simulink model "modelo_planta"  (R2023b)
settings: Solver=VariableStepAuto  StartTime=0.0  StopTime=inf  MaxStep=1e-3  RelTol=1e-3
undefined symbols (not defined in the file): ah_max, at_max, bcx, bcy, bhb, bhd, bhEb, bhm, bhwu, bt, btb, btd, btm, btw, DiscIntNeverNeededParam, g, h_vec_inicial, Hc, ih, it, J_hd_hEb, J_hm_hb, Jtd, Jtm_tb, Kcy, khwu, Ki_h, Ki_t, Kp_h, Kp_t, Kpos_h, Kpos_t, Ktw, lambda, Lh0, lh_0, magnitude, Mc_max, Mc_min, Ms, Mt, P_nom, rhd, rtd, tau_hm, tau_tm, Thb_Max, ThEb_Max, Thm_0, Thm_Max, titahm_0, titatm_0, Ts0, Ts1, Ts2, Ttb_Max, Ttm_0, Ttm_Max, vh_max_unloaded, vh_nom ... (+20)
libraries: simulink x14, vrlib x1, simulink_extras x1, dspnetwork x1
(part 2 of 2)

== stateflow chart modelo_planta/Control Nivel 1 ==
  settings: updateMethod=DISCRETE  sampleTime=Ts1
  state MAQUINA_ESTADOS [parallel]
    settings: executionOrder=1
    state AUTO
      state CICLO_SIMPLE
        entry:
        ciclo_doble = 0;
      state SELECCION_INDICE_INI_1
        entry:
        seleccionando_i(1) = 1;
        seleccionando = 1;
        is_cont = 0;
        during:
        i_ini1 = i_x_cruz;
        is_cont = check_container(i_ini1, yc0_vec);
        exit:
        i_obj_vec(1) = i_ini1;
        seleccionando_i(1) = 0;
      state SELECCION_INDICE_FIN_1
        entry:
        seleccionando_i(2) = 1;
        during:
        i_fin1 = i_x_cruz;
        exit:
        i_obj_vec(2) = i_fin1;
        seleccionando_i(2) = 0;
      state SELECCION_INDICE_INI_2
        entry:
        seleccionando_i(3) = 1;
        is_cont = 0;
        during:
        i_ini2 = i_x_cruz;
        is_cont = check_container(i_ini2, yc0_vec);
        exit:
        i_obj_vec(3) = i_ini2;
        seleccionando_i(3) = 0;
      state AUTO_INIT
        entry:
        modo_auto = 1; modo_manual = 0;
        BRK_t_N1 = 1; BRK_h_N1 = 1;
        x_cmd = 0; y_cmd = 0;
        estado = 1; % Bandera de etapa de movimiento
        i_obj_vec = [0,0,0,0];
        seleccionando_i = [0,0,0,0];
        modo_manual_auto = 0; flag = 0;
      state CICLO_DOBLE
        entry:
        ciclo_doble = 1;
      state SELECCION_INDICE_FIN_2
        entry:
        seleccionando_i(4) = 1;
        during:
        i_fin2 = i_x_cruz;
        exit:
        i_obj_vec(4) = i_fin1;
        seleccionando_i(4) = 0;
      state MANUAL_SIMPLE
        entry:
        modo_manual = 1; modo_auto = 0;
        modo_manual_auto = 1; flag = 0;
        y_handover = y_ref;
        y_cruz = y_ref;
        x_cruz = x_ref;
        during:
        x_cruz = xt_enc;
        y_ref = y_cruz;
        if (TLK == 0)
        y_cruz = max([yc0-offset, min(y_handover, y_cruz)]);
        elseif (TLK == 1)
        y_cruz = max([(yc0+Hc)-offset, min(y_handover, y_cruz)]);
        end
        exit:
        estado = estado + 1;
      state MOVIMIENTO_CURVO
        entry:
        modo_auto = 1;
        modo_manual_auto = 0; flag = 1;
        manual_ok = 0;
        i_usado = 0;
        seleccionando = 0;
        during:
        if (estado == 1) i_usado = i_ini1;
        elseif (estado == 2) i_usado = i_fin1;
        elseif (estado == 3) i_usado = i_ini2;
        elseif (estado == 4) i_usado = i_fin2;
        end
        [x_cmd, y_cmd, manual_ok] = Planificador_Trayectoria...
        (xt_enc, yh_enc, i_usado, yc0_vec, TLK, theta_l);
        x_ref = x_cmd;
        y_ref = y_cmd;
        % Actualizar cruz con referencias
        x_cruz = x_ref;
        y_cruz = y_ref;
      (default) -> MAQUINA_ESTADOS.AUTO.AUTO_INIT
      CICLO_SIMPLE -> MAQUINA_ESTADOS.AUTO.SELECCION_INDICE_INI_1 [order 1] : [rising(BTN_TLK)]
      MAQUINA_ESTADOS.AUTO.AUTO_INIT -> CICLO_SIMPLE
      CICLO_SIMPLE -> CICLO_DOBLE [order 2] : [rising(BTN_Auto)]
      CICLO_DOBLE -> CICLO_SIMPLE [order 2] : [rising(BTN_Auto)]
      MAQUINA_ESTADOS.AUTO.SELECCION_INDICE_INI_1 -> MAQUINA_ESTADOS.AUTO.SELECCION_INDICE_FIN_1 : [rising(BTN_TLK)&& is_cont == 1]
      MAQUINA_ESTADOS.AUTO.SELECCION_INDICE_FIN_1 -> SELECCION_INDICE_INI_2 [order 2] : [rising(BTN_TLK) && ciclo_doble == 1]
      CICLO_DOBLE -> MAQUINA_ESTADOS.AUTO.SELECCION_INDICE_INI_1 [order 1] : [rising(BTN_TLK)]
      MAQUINA_ESTADOS.AUTO.SELECCION_INDICE_FIN_1 -> MOVIMIENTO_CURVO [order 1] : [rising(BTN_TLK) && ciclo_doble == 0]
      MANUAL_SIMPLE -> MAQUINA_ESTADOS.AUTO.AUTO_INIT [order 1] : [TLK == 0 && yh_enc >= (y_handover - 0.1) && estado == 2 && ciclo_doble == 0]
      MANUAL_SIMPLE -> MAQUINA_ESTADOS.AUTO.AUTO_INIT [order 4] : [TLK == 0 && yh_enc >= (y_handover - 0.1) && estado == 4 && ciclo_doble == 1]
      SELECCION_INDICE_INI_2 -> SELECCION_INDICE_FIN_2 : [rising(BTN_TLK) && is_cont == 1 ]
      SELECCION_INDICE_FIN_2 -> MOVIMIENTO_CURVO : [rising(BTN_TLK)]
      MOVIMIENTO_CURVO -> MANUAL_SIMPLE [order 1] : [manual_ok == 1]
      MANUAL_SIMPLE -> MOVIMIENTO_CURVO [order 5] : [TLK == 1 && yh_enc >= (y_handover - 0.1) && estado == 3]
      MANUAL_SIMPLE -> MOVIMIENTO_CURVO [order 3] : [TLK == 0 && yh_enc >= (y_handover - 0.1) && estado == 2]
      MANUAL_SIMPLE -> MOVIMIENTO_CURVO [order 2] : [TLK == 1 && yh_enc >= (y_handover - 0.1) && estado == 1]
    state STOP
      entry:
      x_ref = xt_0; y_ref = yh_0;
      x_cruz = x_ref; y_cruz = y_ref;
      x_cruz_unity = x_ref; y_cruz_unity = y_ref;
      seleccionando = 0;
      vx_cmd = 0; vy_cmd = 0;
      BRK_t_N1 = 0; BRK_h_N1 = 0; % Frenos Cerrados
      modo_manual = 0; modo_auto = 0;
      dead_zone = 0.1; % Zona muerta joystick
      offset = 0.2; % Offset del apoyo
      modo_manual_auto = 0; flag = 0; % Bandera para bumpless transfer
      ciclo_doble = 0;
    state POSICION_SEGURA
      entry:
      x_ref = xt_0; y_ref = yh_0;
      BRK_t_N1 = 1; BRK_h_N1 = 1;
    state ERROR
      entry:
      BRK_t_N1 = 0; BRK_h_N1 = 0;
    state MANUAL
      state MANUAL_INIT [parallel]
        entry:
        % Si quiero mover, abro frenos
        BRK_t_N1 = 1;
        BRK_h_N1 = 1;
        modo_manual = 1;
        settings: executionOrder=1
      state INTEGRACION_JOYSTICK [parallel]
        during:
        % Copiar los movimientos de la cruceta
        x_ref = x_cruz
        y_ref = y_cruz
        % Cuando los índices son diferentes
        if(i_xt_ref ~= i_carro && y_ref<yc0_xtref+1)
        if (TLK == 1)
        y_ref = max([(yc0+Hc)-offset, (yc0_xtref+Hc)+1, min(yh_max, y_ref)]);
        else
        y_ref = max([yc0-offset, yc0_xtref+1, min(yh_max, y_ref)]);
        end
        % Aplico la limitación a la cruceta
        y_cruz = y_ref;
        % Cuando están en el mismo índice
        else
        if (TLK == 1)
        y_ref = max([(yc0+Hc)-offset, min(yh_max, y_ref)]);
        if (sobrecarga == 1)
        % No se puede mover en horizontal
        x_ref = xt_enc;
        % En vertical solo puede moverse hacia abajo
        y_ref = max([(yc0+Hc)-offset, min((yc0+Hc)+offset,y_ref)]);
        end
        else
        y_ref = max([yc0-offset, min(yh_max, y_ref)]);
        end
        end
        % Aplico las limitaciones del modo manual a la cruceta
        x_cruz = x_ref;
        y_cruz = y_ref;
        settings: executionOrder=2
    (default) -> STOP
    STOP -> AUTO [order 1] : [rising(BTN_Auto) && FALLA == 0]
    STOP -> ERROR [order 2] : [FALLA == 1]
    STOP -> MANUAL [order 3] : [rising(BTN_Manual) && FALLA == 0]
    POSICION_SEGURA -> STOP : [abs(xt_enc - x_ref) <= 0.1 && abs(yh_enc - y_ref) <= 0.1 && abs(vt_enc) <= 0.008]
    ERROR -> POSICION_SEGURA : [FALLA == 0 && rising(BTN_Reset)]
    AUTO -> ERROR [order 2] : [FALLA == 1]
    MANUAL -> ERROR [order 1] : [FALLA ==1 || FC_der == 1 || FC_izq == 1 || FC_sup == 1 || FC_inf == 1]
    AUTO -> MANUAL [order 1] : [rising(BTN_Manual) && modo_manual_auto == 0]
    MANUAL -> AUTO [order 3] : [rising(BTN_Auto) && flag == 0]
    MANUAL_SIMPLE -> MANUAL [order 6] : [rising(BTN_Manual) && modo_auto == 0]
    MANUAL -> MOVIMIENTO_CURVO [order 2] : [rising(BTN_Auto) && flag == 1]
    MOVIMIENTO_CURVO -> MANUAL [order 2] : [Joy_XY(1) > dead_zone || Joy_XY(2) > dead_zone || rising(BTN_Manual)]
  state MONITOREO_FISICO [parallel]
    settings: executionOrder=2
    state LIMITE_VEL_CARRO [parallel]
      during:
      factor_x = 1.0;
      dist_dinamica = 3.5 - (0.166 * yh_enc); % Definir zona de frenado (m antes del tope)
      dist_frenado_x = max(2.0, min(3.5, dist_dinamica)); % Saturación por seguridad (2m < x < 10m)
      % Acercándose al Muelle (xt_min)
      if (xt_enc < (xt_min + dist_frenado_x)) && (vx_cmd <= 0)
      factor_x = 0.1;  % 10% de la velocidad
      % Acercándose al Barco (xt_max)
      elseif (xt_enc > (xt_max - dist_frenado_x)) && (vx_cmd >= 0)
      factor_x = 0.1;
      end
      vt_lim = vt_max * factor_x;
      settings: executionOrder=1
    state TWISTLOCKS [parallel]
      settings: executionOrder=2
      state ABRIENDO_TLK
        entry:
        TLK = 0;
        y_start = yh_enc;
        trans_TLK = 1;
        during:
        vh_lim = 0.5;
        m_est = max(Ms, Fhw * 2 / g);
        y_ref = yh_enc + 0.5;
        x_ref = xt_enc;
        % Coordinar cruz con referencias
        y_cruz = y_ref;
        x_cruz = x_ref;
      state VACIO
        entry:
        TLK = 0;
        m_est = Ms;
        vh_lim = vh_max_unloaded;
        sobrecarga = 0;
        trans_TLK = 0;
      state CERRANDO_TLK
        entry:
        TLK = 1;
        y_start = yh_enc;
        trans_TLK = 1;
        during:
        vh_lim = 0.5;
        m_est = max(Ms, (Fhw * 2 / g));
        y_ref = yh_enc + 0.1;
        x_ref = xt_enc;
        % Coordinar cruz con referencias
        y_cruz = y_ref;
        x_cruz = x_ref;
      state CARGADO
        entry:
        trans_TLK = 0;
        v_potencia = P_nom / (m_est * g);
        vh_lim = min(vh_max_unloaded, max(vh_nom, v_potencia));
        % Sobrecarga (margen 100kg)
        if (m_est > (Ms + Mc_max + 100))
        sobrecarga = 1;
        vh_lim = 0.1;
        vt_lim = 0;
        end
        during:
        m_est = max(Ms, (Fhw * 2 / g));
      (default) -> VACIO
      ABRIENDO_TLK -> VACIO : [Fhw >= (Ms*g/2*0.8) && (yh_enc - y_start) > 0.3 &&  xt_enc <= x_ref + 0.1]
      VACIO -> CERRANDO_TLK : [rising(BTN_TLK) == 1 && Fhw < (Ms*g/2*0.8) && ((i_carro<13 && yc0>0 ) || (i_carro>13 && i_carro<33 && yc0>-18))]
      CARGADO -> ABRIENDO_TLK : [falling(BTN_TLK) == 1 && Fhw < (m_est*g/2*0.8)]
      CERRANDO_TLK -> CARGADO : [Fhw > (Ms*g/2 * 1.2) && (yh_enc - y_start) > 0.3 && xt_enc <= x_ref +0.1]
  state MODO_AUTO_CUADRADO [parallel] [commented out]
    state AUTO_INIT [commented out]
      entry:
      modo_auto = 1; modo_manual = 0;
      BRK_t_N1 = 1; BRK_h_N1 = 1;
      x_cmd = 0; y_cmd = 0;
      flag = 0;
    state SELECCION_INDICE_FIN_1 [commented out]
      entry:
      i_fin1 = 20;
      exit:
      flag = 1;
    state SELECCION_INDICE_INI_1 [commented out]
      entry:
      i_ini1 = 5;
      ini = check_container(i_ini1, yc0_vec);
    state MODO_MANUAL [commented out]
      entry:
      modo_manual = 1;
      v_max_ref = 3;     % Vel. de la referencia
      y_handover = y_ref;
      during:
      Joy_CMD_Y = Joy_XY(2);
      if abs(Joy_CMD_Y) < dead_zone
      vy_cmd = 0;
      else
      vy_cmd = Joy_CMD_Y * v_max_ref;
      end
      y_ref = y_ref + vy_cmd * Ts1;
      if (TLK == 0)
      y_ref = max([yc0-offset, min(y_handover, y_ref)]);
      elseif (TLK == 1)
      y_ref = max([(yc0+Hc)-offset, min(y_handover, y_ref)]);
      end
      exit:
      modo_auto = modo_auto + 1;
    state BUSCAR_Y_MOVER_Y1 [commented out]
      entry:
      BRK_t_N1 = 1; BRK_h_N1 = 1;
      if modo_auto == 0
      if i_carro < i_ini1
      max_h = max(yc0_vec(i_carro : i_ini1));
      else
      max_h = max(yc0_vec(i_ini1 : i_carro));
      end
      y_ref = max_h + 2; % 2m de h_max
      elseif modo_auto == 1
      if i_carro < i_fin1
      max_h = max(yc0_vec(i_carro : i_fin1));
      else
      max_h = max(yc0_vec(i_fin1 : i_carro));
      end
      y_ref = max_h + 2 + Hc; % 2m de h_max
      end
    state MOVER_X1 [commented out]
      entry:
      if modo_auto == 0
      if i_carro < i_ini1
      x_ref = xt_min + (i_ini1-1) * Wc - Wc/2;
      elseif i_carro > i_ini1
      x_ref = xt_min + (i_ini1+1) * Wc - Wc/2;
      end
      elseif modo_auto == 1
      if i_carro < i_fin1
      x_ref = xt_min + (i_fin1-2) * Wc - Wc/2;
      elseif i_carro > i_fin1
      x_ref = xt_min + (i_fin1+2) * Wc - Wc/2;
      end
      end
    state BAJAR_SPREADER1 [commented out]
      entry:
      if modo_auto == 0
      y_ref = yc0_vec(i_ini1) + 2;
      elseif modo_auto == 1
      y_ref = (yc0_vec(i_fin1) + Hc) +2
      end
      y_handover = y_ref;
    state MOVER_X2 [commented out]
      entry:
      if modo_auto == 0
      x_ref = xt_min + i_ini1 * Wc - Wc/2;
      elseif modo_auto == 1
      x_ref = xt_min + i_fin1 * Wc - Wc/2;
      end
    (default) -> MODO_AUTO_CUADRADO.AUTO_INIT [commented out]
    MODO_AUTO_CUADRADO.SELECCION_INDICE_INI_1 -> MODO_AUTO_CUADRADO.SELECCION_INDICE_FIN_1 [commented out] : [rising(BTN_Auto) && ini == 1]
    MODO_AUTO_CUADRADO.AUTO_INIT -> MODO_AUTO_CUADRADO.SELECCION_INDICE_INI_1 [commented out] : [rising(BTN_Auto)]
    MODO_AUTO_CUADRADO.SELECCION_INDICE_FIN_1 -> BUSCAR_Y_MOVER_Y1 [commented out] : [rising(BTN_Auto)]
    MODO_MANUAL -> MODO_AUTO_CUADRADO.AUTO_INIT [commented out] : [TLK == 0 && yh_enc >= (y_handover - 0.1) && modo_auto == 2]
    MODO_MANUAL -> BUSCAR_Y_MOVER_Y1 [commented out] : [TLK == 1 && yh_enc >= (y_handover - 0.1) && modo_auto == 0]
    BUSCAR_Y_MOVER_Y1 -> MOVER_X1 [commented out] : [yh_enc > y_ref || abs(yh_enc - y_ref) <= 3]
    BAJAR_SPREADER1 -> MODO_MANUAL [commented out] : [abs(yh_enc - y_ref) <= 0.1]
    MOVER_X2 -> BAJAR_SPREADER1 [commented out] : [abs(xt_enc - x_ref) <= 0.1]
    MOVER_X1 -> MOVER_X2 [commented out] : [abs(xt_enc - x_ref) <= 2]
  state INIDICES_Y_PERFIL [parallel]
    settings: executionOrder=3
    state ACTUALIZAR_PERFIL_ALTURAS [parallel]
      entry:
      yc0_xtref = 0;
      yc0 = 0;
      yc0_vec_output = yc0_vec;
      h_vec_output = h_vec;
      TLK_anterior = 0;
      during:
      yc0_xtref = yc0_vec(i_xt_ref); % Obtengo altura donde esta la referencia
      yc0_vec_output(i_lidar) = h_vec(i_lidar); % Actualizo perfil con la medición real
      %Detecto si se ha abierto o cerrado TLK
      TLK_rise  = (TLK_anterior == 0) && (TLK == 1);
      TLK_fall  = (TLK_anterior == 1) && (TLK == 0);
      % Si agarré un container, hay que bajar el perfil
      if(TLK_rise)
      h_vec_output(i_carro) = h_vec(i_carro)-Hc;
      yc0_vec_output(i_carro) = yc0_vec(i_carro)-Hc;
      %Si solté un container, hay que aumentar el perfil
      elseif(TLK_fall)
      h_vec_output(i_carro) = h_vec(i_carro)+Hc;
      yc0_vec_output(i_carro) = yc0_vec(i_carro)+Hc;
      end
      yc0 = yc0_vec_output(i_carro);
      TLK_anterior = TLK;
      settings: executionOrder=2
    state CALCULO_INDICES [parallel]
      entry:
      i_carro = 0;
      i_lidar = 0;
      i_xt_ref = 0;
      i_x_cruz = 0;
      during:
      i_carro = floor((xt_enc - xt_min)/Wc) + 1;
      i_carro = min(max(i_carro, 1), 33);
      i_lidar = floor((xt_enc+x_LIDAR-xt_min)/Wc)+1;
      i_lidar = min(max(i_lidar,1),33);
      i_xt_ref = floor((x_ref - xt_min)/Wc) + 1;
      i_xt_ref = min(max(i_xt_ref, 1), 33);
      i_x_cruz = floor((x_cruz - xt_min)/Wc) + 1;
      i_x_cruz = min(max(i_x_cruz, 1), 33);
      settings: executionOrder=1
  state HAY_CONTAINER_ABAJO [parallel] [commented out]
    entry:
    hay_container = 0;
    during:
    if(i_carro<13 && yc0>0)
    hay_container = 1;
    elseif(i_carro>13 && i_carro<33 &&yc0>-18)
    hay_container = 1;
    else
    hay_container=0;
    end
  note: El orden es importante! Si no van en orden los bloques no funcionan:
      | Maquina estados
      | Monitoreo fisico
      | Indices y perfil (¡siempre al último!)
  state MANEJO_CRUCETA [parallel]
    settings: executionOrder=4
    state INPUT_JOYSTICK [parallel]
      entry:
      v_max_ref = 8;     % Vel. de la referencia
      during:
      Joy_CMD_X = Joy_XY(1);
      Joy_CMD_Y = Joy_XY(2);
      if abs(Joy_CMD_X) < dead_zone
      vx_cmd = 0;
      else
      vx_cmd = Joy_CMD_X * v_max_ref;
      end
      if abs(Joy_CMD_Y) < dead_zone
      vy_cmd = 0;
      else
      vy_cmd = Joy_CMD_Y * v_max_ref;
      end
      if (trans_TLK == 1)
      vx_cmd = 0;
      vy_cmd = 0;
      end
      settings: executionOrder=1
    state ACTUALIZAR_CRUCETA [parallel]
      during:
      % Actualizar posición x de la cruceta
      x_cruz = x_cruz + vx_cmd * Ts1;
      % Actualizar posición y de la cruceta
      y_cruz = y_cruz + vy_cmd * Ts1;
      % Limitar en x
      x_cruz = max(xt_min, min(xt_max, x_cruz));
      % Limitar en y
      y_cruz = max(yh_min, min(yh_max, y_cruz));
      if seleccionando == 0
      x_cruz_unity = x_cruz;
      y_cruz_unity = y_cruz;
      else
      x_cruz_unity = xt_min + i_x_cruz * Wc - Wc/2;
      y_cruz_unity = yh_min;
      end
      settings: executionOrder=2
  data: i_pos function_input; y0_vec function_input; hay_container function_output; x_real function_input; y_real function_input; i_ref function_input; y0_vec function_input; twistlock function_input; tita_l function_input; x_ref_out function_output; y_ref_out function_output; listo_para_manual function_output; xt_enc function_input; yh_enc function_input; i_xt_ref function_input; h_vec function_input; TLK function_input; x_ref_out function_output; y_ref_out function_output; listo_para_manual function_output; vt_enc input; Fhw input size=1; BTN_TLK input size=1; m_est output size=1; vh_lim output size=1; vh_max_unloaded parameter size=1; P_nom parameter size=1; g parameter size=1; Ms parameter size=1; Joy_XY input; BTN_Manual input size=1; BTN_Auto input size=1; BTN_Reset input size=1; FC_der input size=1; FC_sup input size=1; FC_izq input size=1; FC_inf input size=1; xt_enc input size=1; yh_enc input size=1; FALLA input size=1; x_ref output size=1; y_ref output size=1; BRK_h_N1 output size=1; BRK_t_N1 output size=1; Ts1 parameter size=1; xt_0 parameter size=1; yh_0 parameter size=1; xt_max parameter size=1; xt_min parameter size=1; yh_max parameter size=1; vt_max parameter size=1; vt_lim output size=1; vh_nom parameter size=1; Mc_max parameter size=1; TLK output size=1; Wc parameter; x_LIDAR parameter; yc0 output; Hc parameter; yc0_vec input; yc0_vec_output output; h_vec input; h_vec_output output; i_fin1 local; i_xt_ref local; TLK_rise local; TLK_fall local; i_lidar local; y_start local; i_carro local; x_cmd local; y_cmd local; dist_dinamica local; dist_frenado_x local; trans_TLK local; sobrecarga local; yc0_xtref local; TLK_anterior local; v_potencia local; v_max_ref local; Joy_CMD_Y local; Joy_CMD_X local; dead_zone local; factor_x local; vx_cmd local; i_ini1 local; vy_cmd local; offset local; manual_ok local; y_handover local; flag local; i_fin2 local; i_ini2 local; i_usado local; modo_manual_auto local; modo_manual output; modo_auto output; theta_l input; estado local; ciclo_doble output; yh_min parameter; i_x_cruz local; is_cont local; seleccionando_i output; i_obj_vec output; seleccionando local; y_cruz local; x_cruz local; x_cruz_unity output; y_cruz_unity output
  function hay_container  = check_container(i_pos, y0_vec):
    | function hay_container  = check_container(i_pos, y0_vec)
    |    if(i_pos<13 && y0_vec(i_pos)>0)
    |        hay_container = 1;
    |    elseif(i_pos>13 && i_pos<33 && y0_vec(i_pos)>-18)
    |        hay_container = 1;
    |    else
    |        hay_container = 0;
    |    end
    | end
  function [x_ref_out, y_ref_out, listo_para_manual] = Planificador_Trayectoria...:
    | function [x_ref_out, y_ref_out, listo_para_manual] = Planificador_Trayectoria...
    |     (x_real, y_real, i_ref, y0_vec, twistlock, tita_l)
    |     
    |     % 1. SISTEMA DE MEMORIA (LATCH / HISTÉRESIS)
    |     % Estas variables recuerdan el estado entre ejecuciones para evitar
    |     % comportamientos erráticos ("twitching") cuando las señales oscilan en el umbral.
    |     persistent fase_final_latched; % Flag: true = yendo al objetivo real, false = esperando en objetivo falso
    |     persistent last_target_idx;    % Memoria del último destino solicitado por el usuario
    |     
    |     % Inicialización en el primer ciclo de reloj
    |     if isempty(fase_final_latched)
    |         fase_final_latched = false;
    |         last_target_idx = -1;
    |     end
    |     
    |     % RESETEO DE ESTADO:
    |     % Si el operador cambia el destino (ej. de índice 16 a 20),
    |     % forzamos el reinicio de la lógica de aproximación.
    |     if i_ref ~= last_target_idx
    |         fase_final_latched = false;
    |         last_target_idx = i_ref;
    |     end
    | 
    |     % 2. CONFIGURACIÓN Y PARÁMETROS DE SEGURIDAD
    |     % Márgenes geométricos para evitar colisiones físicas
    |     MARGEN_Y_SEG = 2.5;        % Altura extra sobre obstáculos durante el viaje
    |     MARGEN_HOVER = 2.5;        % Altura final sobre el objetivo (punto de entrega)
    |     GAP_X_SEGURIDAD = 1.5;     % Distancia de frenado antes de chocar lateralmente
    |     PENDIENTE_SUBIDA = 0.25;   % Relación de ascenso (1 m subida cada 4 m avance)
    |     
    |     % Definimos una ventana para la estabilidad del péndulo.
    |     % Para entrar a la zona de precisión, el ángulo debe ser muy bajo (< 1.0°)
    |     % Para salir (abortar), el ángulo debe ser muy alto (> 2.0°)
    |     % Esto evita que el sistema oscile entre modos si la variación del ángulo es pequeña.
    |     UMBRAL_ENTRADA = 0.0175; % ~1.0 grado
    |     UMBRAL_SALIDA  = 0.0349; % ~2.0 grados
    |     
    |     % COMPENSACIÓN DE ALTURA DE CARGA
    |     % Si llevamos contenedor (TLK=1), todo el sistema debe subir más
    |     % para compensar la altura física del objeto colgado (Hc).
    |     if twistlock == 1
    |         H_extra = Hc; 
    |     else
    |         H_extra = 0;  % Spreader vacío
    |     end
    |     
    |     % 3. MAPEO Y GESTIÓN DE OBJETIVOS
    |     N = length(y0_vec); 
    |     i_objetivo_final = i_ref;
    |     
    |     % Conversión: Posición actual (metros) -> Índice del mapa
    |     i_actual = floor((x_real - xt_min)/Wc) + 1;
    |     i_actual = min(max(i_actual, 1), N); % Saturación para no salir del vector
    |     
    |     % --- ESTRATEGIA DE OBJETIVO FALSO (ANTI-SWAY) ---
    |     % Definimos un "punto de espera" antes del destino real.
    |     % La grúa viajará rápido hasta aquí y esperará a que el balanceo se disipe.
    |     L_cable = 40.0 - y_real;
    |     
    |     % DIST_TRIGGER Dinámico 
    |     DIST_TRIGGER = 0.1 * L_cable; % Metros antes del objetivo falso para evaluar transición
    |     
    |     % Saturación para seguridad
    |     DIST_TRIGGER = max(0.1, min(5.0, DIST_TRIGGER));
    |     
    |     offset_idx = 1;   % Cantidad de celdas de anticipación
    |     
    |     % Determinar dirección de movimiento para saber de qué lado poner el falso
    |     dir_mov = sign(i_objetivo_final - i_actual);
    |     if dir_mov == 0, dir_mov = 1; end
    |     
    |     i_target_falso = i_objetivo_final - (dir_mov * offset_idx);
    |     
    |     % Cálculo del centro físico (en metros) del objetivo falso
    |     x_falso_m = xt_min + i_target_falso * Wc - Wc/2;
    |     
    |     % 4. LÓGICA DE TRANSICIÓN DE ESTADOS (MAQUINA DE ESTADOS)
    |     
    |     % A. Verificación de posición: ¿Ya llegamos al punto de trigger?
    |     distancia_ok = false;
    |     if dir_mov > 0 % Viajando a derecha
    |         if x_real >= (x_falso_m - DIST_TRIGGER)
    |             distancia_ok = true;
    |         end
    |     else % Viajando a izquierda
    |         if x_real <= (x_falso_m + DIST_TRIGGER)
    |             distancia_ok = true;
    |         end
    |     end
    |     
    |     % B. Lógica del Latch (Cerrojo)
    |     if fase_final_latched == false
    |         % ESTADO: APROXIMACIÓN (Viajando al objetivo falso)
    |         % Solo permitimos pasar a la fase final si estamos cerca Y el péndulo está quieto.
    |         if distancia_ok && (abs(tita_l) < UMBRAL_ENTRADA)
    |             fase_final_latched = true;
    |         end
    |     else
    |         % ESTADO: FASE FINAL (Posicionamiento fino en objetivo real)
    |         % Ya estamos comprometidos. Solo abortamos si la oscilación se vuelve peligrosa.
    |         if abs(tita_l) > UMBRAL_SALIDA
    |             fase_final_latched = false; % Abortar maniobra, volver a esperar
    |         end
    |     end
    | 
    |     % C. Selección de Referencia según el estado del Latch
    |     if fase_final_latched
    |         i_target_eff = i_objetivo_final; % Ir al hueco final
    |         fase_aproximacion = false; 
    |     else
    |         i_target_eff = i_target_falso;   % Quedarse esperando afuera
    |         fase_aproximacion = true;  
    |     end
    |     
    |     % Conversión final Índice -> Metros para el controlador de posición
    |     x_target_cmd = xt_min + i_target_eff * Wc - Wc/2;
    |     
    |     % 5. GENERACIÓN DE TRAYECTORIA SEGURA
    |     x_ref_out = x_target_cmd; 
    |     
    |     % PARTE A: ESCANEO DE PAREDES (BLOQUEO DE MOVIMIENTO X)
    |     % Proyectamos una diagonal desde la posición actual. Si algún obstáculo
    |     % interrumpe esa diagonal, limitamos el movimiento X.
    |     for k = i_actual : dir_mov : i_target_eff
    |         if k < 1 || k > N, continue; end
    |         
    |         h_obs = y0_vec(k);
    |         % Altura mínima requerida para pasar (Obstáculo + Margen + Carga)
    |         techo_nec = h_obs + MARGEN_Y_SEG + H_extra;
    |         
    |         x_centro_celda = xt_min + (k - 1) * Wc + Wc/2;
    |         dist_al_centro = abs(x_centro_celda - x_real);
    |         
    |         % Proyección: Altura actual + (Distancia * Pendiente)
    |         h_proyectada = y_real + (dist_al_centro * PENDIENTE_SUBIDA);
    |         
    |         % Si mi proyección choca con el techo necesario -> FRENAR X
    |         if h_proyectada < techo_nec    
    |             mitad_ancho_real = Wc / 2;
    |             if dir_mov > 0 
    |                 x_borde_fisico = x_centro_celda - mitad_ancho_real;
    |                 x_bloqueo = x_borde_fisico - GAP_X_SEGURIDAD;
    |                 x_ref_out = max(x_real, x_bloqueo); % Saturar referencia
    |             else 
    |                 x_borde_fisico = x_centro_celda + mitad_ancho_real;
    |                 x_bloqueo = x_borde_fisico + GAP_X_SEGURIDAD;
    |                 x_ref_out = min(x_real, x_bloqueo);
    |             end
    |             break; % El primer obstáculo manda
    |         end
    |         if k == i_target_eff, break; end
    |     end
    |     
    |     % PARTE B: ESCANEO DE TECHO (CONTROL DE ALTURA Y)
    |     % Calculamos qué tan bajo podemos ir sin chocar con nada en el camino restante.
    |     
    |     h_destino_final = y0_vec(i_objetivo_final);
    |     y_meta_hover = h_destino_final + MARGEN_HOVER + H_extra;
    |     
    |     % Verificar si el carro está alineado físicamente con el destino X
    |     sobre_destino_x = abs(x_real - x_target_cmd) < 0.5;
    |     
    |     % Buscar el obstáculo más alto entre mi posición y el destino efectivo
    |     i_start = min(i_actual, i_target_eff);
    |     i_end   = max(i_actual, i_target_eff);
    |     
    |     h_max_camino = 0;
    |     for k = i_start : i_end
    |         if y0_vec(k) > h_max_camino
    |             h_max_camino = y0_vec(k);
    |         end
    |     end
    |     
    |     y_techo_dinamico = h_max_camino + MARGEN_Y_SEG + H_extra;
    |     
    |     % DECISIÓN FINAL DE BAJADA
    |     % Condición estricta para bajar al Hover:
    |     % 1. Angulo estable (< 1.0 grado)
    |     % 2. Posición X alineada con el destino
    |     % 3. Fase final activada (no estamos persiguiendo objetivo falso)
    |     sway_para_bajada = abs(tita_l) < UMBRAL_ENTRADA; 
    |     
    |     if sobre_destino_x && (~fase_aproximacion) && sway_para_bajada
    |         % Aterrizaje permitido: Bajar a altura de entrega
    |         y_ref_out = y_meta_hover;
    |     else
    |         % Aterrizaje prohibido: Mantenerse sobre el "techo dinámico" más alto
    |         y_ref_out = max(y_meta_hover, y_techo_dinamico);
    |     end
    |     
    |     % 6. SEÑAL DE LISTO PARA MANUAL
    |     x_destino_meters = xt_min + i_ref * Wc - Wc/2;
    |     dist_error_x = abs(x_real - x_destino_meters);
    |     dist_error_y = abs(y_real - y_meta_hover);
    |     
    |     % Solo entregamos el control si estamos en posición y estables
    |     if (dist_error_x < 0.1) && (dist_error_y < 0.1) && (~fase_aproximacion) && sway_para_bajada
    |         listo_para_manual = 1;
    |     else
    |         listo_para_manual = 0;
    |     end
    | end
  function [x_ref_out, y_ref_out, listo_para_manual] = Planificador_Trayectoria_Antiguo(...:
    | function [x_ref_out, y_ref_out, listo_para_manual] = Planificador_Trayectoria_Antiguo(...
    |     xt_enc, yh_enc, i_xt_ref, h_vec, TLK)
    | 
    |     % SEGURIDAD
    |     MARGEN_Y_SEG = 2.0;        
    |     MARGEN_HOVER = 2.0;        
    |     GAP_X_SEGURIDAD = 2.5;     
    |     PENDIENTE_SUBIDA = 0.25;
    | 
    |     % CÁLCULO DE OFFSET VERTICAL
    |     if TLK == 1
    |         H_extra = Hc; % Si llevo carga, debo estar más alto
    |     else
    |         H_extra = 0;  % Si voy vacío, el spreader es el límite
    |     end
    |     
    |     % SATURACIÓN DE ENTRADAS
    |     N = length(h_vec); 
    |     i_objetivo_final = i_xt_ref;
    | 
    |     % LÓGICA DE MAPEO
    |     i_actual = floor((xt_enc - xt_min)/Wc) + 1;
    |     i_actual = min(max(i_actual, 1), N);
    | 
    |     % GESTIÓN DEL OBJETIVO FALSO (ANTI-SWAY DINÁMICO)
    |     % Parámetro de sintonía fina
    |     DIST_TRIGGER = 2; 
    | 
    |     % 1. Definir Offset de índices (Dónde ponemos el señuelo)
    |     if TLK == 1
    |         offset_idx = 2; % Cargado: Frenamos antes
    |     else
    |         offset_idx = 1; % Vacío: Frenamos más cerca
    |     end
    |     % 2. Calcular Dirección y el Índice del Objetivo Falso
    |     dir_mov = sign(i_objetivo_final - i_actual);
    |     if dir_mov == 0, dir_mov = 1; end
    |     
    |     i_target_falso = i_objetivo_final - (dir_mov * offset_idx);
    | 
    |     % 3. Calcular posición física (metros) del Objetivo Falso
    |     x_falso_m = xt_min + (i_target_falso-1) * Wc - Wc/2;
    | 
    |     % 4. Lógica de Transición por Cruce de Umbral
    |     cruce_exitoso = false;
    |     
    |     if dir_mov > 0 % Yendo a la DERECHA (Indices crecen)
    |         % El trigger está A LA IZQUIERDA del falso objetivo
    |         if xt_enc >= (x_falso_m - DIST_TRIGGER)
    |             cruce_exitoso = true;
    |         end
    |     else % Yendo a la IZQUIERDA (Indices decrecen)
    |         % El trigger está A LA DERECHA del falso objetivo
    |         if xt_enc <= (x_falso_m + DIST_TRIGGER)
    |             cruce_exitoso = true;
    |         end
    |     end
    | 
    |     % 5. Selección del Objetivo Efectivo
    |     if cruce_exitoso
    |         % Ya pasamos el punto de no retorno -> Vamos al REAL
    |         i_target_eff = i_objetivo_final;
    |         fase_aproximacion = false; % Habilitamos precisión final
    |     else
    |         % Aún no llegamos al trigger -> Perseguimos al FALSO
    |         i_target_eff = i_target_falso;
    |         fase_aproximacion = true;  % Mantenemos velocidad
    |     end
    |     
    |     x_target_cmd = xt_min + i_target_eff * Wc - Wc/2;
    | 
    |     % PLANIFICACIÓN DE TRAYECTORIA SEGURA
    |     x_ref_out = x_target_cmd; 
    | 
    |     % A. ESCANEO DE PAREDES (SUBIDA)
    |     for k = i_actual : dir_mov : i_target_eff
    |         if k < 1 || k > N, continue; end
    |         
    |         h_obs = h_vec(k);
    |         techo_nec = h_obs + MARGEN_Y_SEG + H_extra;
    |         
    |         x_centro_celda = xt_min + (k - 1) * Wc + Wc/2;
    |         dist_al_centro = abs(x_centro_celda - xt_enc);
    |         
    |         % Proyección diagonal
    |         h_proyectada = yh_enc + (dist_al_centro * PENDIENTE_SUBIDA);
    |         
    |         if h_proyectada < techo_nec    
    |             % Frenado de Precisión (Siempre aplica para no chocar lateralmente)
    |             mitad_ancho_real = Wc / 2;
    |             if dir_mov > 0 
    |                 x_borde_fisico = x_centro_celda - mitad_ancho_real;
    |                 x_bloqueo = x_borde_fisico - GAP_X_SEGURIDAD;
    |                 x_ref_out = max(xt_enc, x_bloqueo);
    |             else 
    |                 x_borde_fisico = x_centro_celda + mitad_ancho_real;
    |                 x_bloqueo = x_borde_fisico + GAP_X_SEGURIDAD;
    |                 x_ref_out = min(xt_enc, x_bloqueo);
    |             end
    |             break; 
    |         end
    |         if k == i_target_eff, break; end
    |     end
    |     
    |   % B. ESCANEO DE TECHO (BAJADA)
    |     h_destino_final = h_vec(i_objetivo_final);
    |     y_meta_hover = h_destino_final + MARGEN_HOVER + H_extra;
    |     sobre_destino_x = abs(xt_enc - x_target_cmd) < 0.5;
    |     
    |     i_start = min(i_actual, i_target_eff);
    |     i_end   = max(i_actual, i_target_eff);
    |     
    |     h_max_camino = 0;
    |     for k = i_start : i_end
    |         if h_vec(k) > h_max_camino
    |             h_max_camino = h_vec(k);
    |         end
    |     end
    |     
    |     y_techo_dinamico = h_max_camino + MARGEN_Y_SEG + H_extra;
    | 
    |     % Solo permitimos ignorar el techo dinámico y bajar al hover
    |     % si estamos en el destino X Y ADEMÁS ya no es el objetivo falso.
    |   
    |     if sobre_destino_x && (~fase_aproximacion)
    |         % Estoy en el objetivo REAL. Puedo bajar.
    |         y_ref_out = y_meta_hover;
    |     else
    |         % Estoy viajando o estoy sobre el objetivo falso.
    |         % DEBO respetar la altura del obstáculo debajo de mí.
    |         y_ref_out = max(y_meta_hover, y_techo_dinamico);
    |     end
    |     
    |     % SEÑAL DE ALCANCÉ OBJETIVOS
    |     x_destino_meters = xt_min + i_xt_ref * Wc - Wc/2;
    |     dist_error_x = abs(xt_enc - x_destino_meters);
    |     dist_error_y = abs(yh_enc - y_meta_hover);
    |     
    |     if (dist_error_x < 0.1) && (dist_error_y < 0.1) && (~fase_aproximacion)
    |         listo_para_manual = 1;
    |     else
    |         listo_para_manual = 0;
    |     end
    | end

== stateflow chart modelo_planta/Control Nivel 0 ==
  state SISTEMA_OK
    entry:
    BRK_hE_N0 = 1; BRK_t_N0 = 1;
    FALLA = 0;
  state FALLA_CARRO
    entry:
    BRK_hE_N0 = 1; BRK_t_N0 = 0;
    FALLA = 1;
  state EMERGENCIA
    entry:
    BRK_hE_N0 = 0; BRK_t_N0 = 0;
    FALLA = 1;
  state FALLA_IZAJE
    entry:
    BRK_hE_N0 = 0; BRK_t_N0 = 1;
    FALLA = 1;
  (default) -> SISTEMA_OK
  SISTEMA_OK -> FALLA_IZAJE [order 3] : [FCE_sup == 1 || FCE_inf == 1 || abs(vh_enc) > (1.15 * vh_max_unloaded) ]
  SISTEMA_OK -> FALLA_CARRO [order 2] : [FCE_izq == 1 || FCE_der == 1]
  SISTEMA_OK -> EMERGENCIA [order 1] : [BTN_emerg == 1]
  data: BTN_emerg input size=1; FCE_der input size=1; FCE_sup input size=1; vh_enc input size=1; FALLA output size=1; FCE_izq input size=1; FCE_inf input size=1; BRK_hE_N0 output size=1; BRK_t_N0 output size=1; vh_max_unloaded parameter size=1
